simulink model "SMC1"  (R2018b)
settings: Solver=VariableStepAuto  StartTime=0.0  StopTime=20  MaxStep=0.001  RelTol=1e-3  EnableMultiTasking=on
settings Model: Creator=omid_zandi  LastModifiedBy=Arash
settings OptimizationCC: LifeSpan=inf
settings DebuggingCC: SFUnexpectedBacktrackingDiag=warning  SFNoUnconditionalDefaultTransitionDiag=warning
settings SFSimCC: SimUseLocalCustomCode=off
settings RTWCC: RTWUseLocalCustomCode=off
settings CodeAppCC: StateflowObjectComments=on
settings GRTTargetCC: TargetLangStandard=C89/C90 (ANSI)  GeneratePreprocessorConditionals=Disable all
settings ConfigComp: CovMetricSettings=dw  CovHtmlReporting=on  CovSaveCumulativeToWorkspaceVar=on  CovSaveSingleToWorkspaceVar=on  CovExternalEMLEnable=off

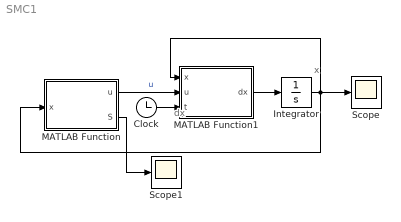
== system SMC1 ==
  note: dx
  note: x
  Clock : Clock
  Integrator : Integrator  InitialCondition=randn(2,1)*10
  MATLAB Function : MATLAB Function  TreatAsAtomicUnit=on
  MATLAB Function1 : MATLAB Function  TreatAsAtomicUnit=on
  Scope : Scope
  Scope1 : Scope
  wires:
  Integrator/1 -> MATLAB Function1/1(x), MATLAB Function/1(x), Scope/1
  MATLAB Function1/1(dx) -> Integrator/1
  Clock/1 -> MATLAB Function1/3(t)
  MATLAB Function/2(S) -> Scope1/1
  MATLAB Function/1(u) -> MATLAB Function1/2(u)  "u"

== matlab function SMC1/MATLAB Function1 ==
  data: x input; dx output; u input; t input
function dx = fcn(x , u , t)
%#codegen
dx = zeros(2,1);
dx(1) = x(2) + x(1)^2; 
a = 1 + exp(-t);
dx(2) =   a *x(2)*x(1)^2 + u;

== matlab function SMC1/MATLAB Function ==
  data: x input; u output; S output
function [u , S] = fcn(x)
k = 4;
eta = 4;
S = x(2) + k * x(1) + x(1)^2 ;
F = abs(x(2)) * (2 * x(1)^2 + k + 2*abs(x(1))); 
u = -(F + eta) * sign(S);
